simulink model "ManipulatorTrajectoryPlanning_Randomized"  (R2023b)
settings: Solver=VariableStepAuto  StartTime=0.0  StopTime=5  RelTol=1e-3
model workspace (MAT data in the model file):
  dq0 = [0; 0; 0; 0; 0; 0; 0; 0; 0]
  q0 = [0; 3.14159265359; 3.14159265359; 0; 0; 0; 0; 0; 0]
  robotToTest : robotics.RigidBodyTree (value not decoded)
symbols that are objects in the model workspace (value not decoded): robotToTest
undefined symbols (not defined in the file): X, Y, Z
libraries: sm_lib x140, nesl_utility x23, robotcorelib x1
(part 1 of 3)
settings Model: Creator=callie  LastModifiedBy=callie
settings OptimizationCC: ReuseModelBlockBuffer=off

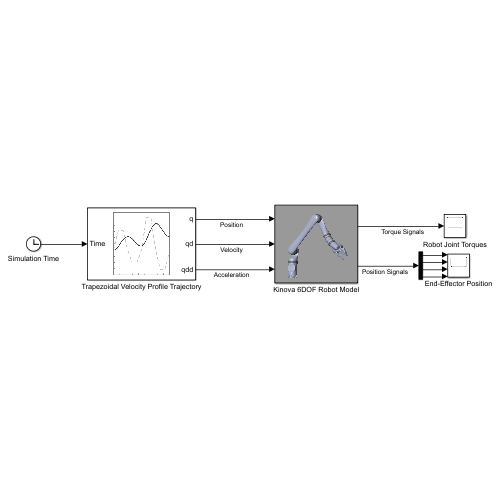
[thumbnail: Simulink's stored preview of the top-level diagram]
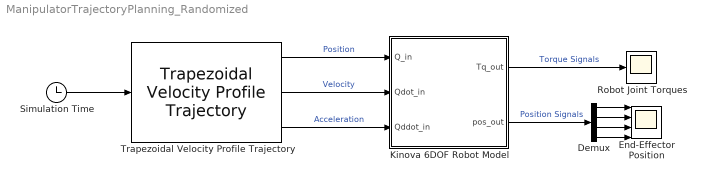
== system ManipulatorTrajectoryPlanning_Randomized ==
  Demux : Demux
  End-Effector Position : Scope  NumInputPorts=4
  Kinova 6DOF Robot Model : Subsystem
      mask Display: image('fullrobot.png'); % Use "Edit Image" on toolstrip to change.
  Robot Joint Torques : Scope
  Simulation Time : Clock
  Trapezoidal Velocity Profile Trajectory : robotcorelib/Trapezoidal Velocity Profile Trajectory  WaypointSource=Internal  Waypoints=[robotToTest.homeConfiguration robotToTest.randomConfiguration robotToTest.randomConfiguration]  NumParams=1  Parameter1=End Time  Parameter2=End Time  ParameterSource=Internal  PeakVelocity=[ 2; 2 ]  Acceleration=[ 1; 2 ]  EndTime=3  AccelTime=[ 1; 2 ]  SimulateUsing=Interpreted execution
  wires:
  Simulation Time/1 -> Trapezoidal Velocity Profile Trajectory/1
  Trapezoidal Velocity Profile Trajectory/1 -> Kinova 6DOF Robot Model/1(Q_in)  "Position"
  Trapezoidal Velocity Profile Trajectory/2 -> Kinova 6DOF Robot Model/2(Qdot_in)  "Velocity"
  Trapezoidal Velocity Profile Trajectory/3 -> Kinova 6DOF Robot Model/3(Qddot_in)  "Acceleration"
  Kinova 6DOF Robot Model/1(Tq_out) -> Robot Joint Torques/1  "Torque Signals"
  Kinova 6DOF Robot Model/2(pos_out) -> Demux/1  "Position Signals"
  Demux/1 -> End-Effector Position/1
  Demux/2 -> End-Effector Position/2
  Demux/3 -> End-Effector Position/3
  Demux/4 -> End-Effector Position/4

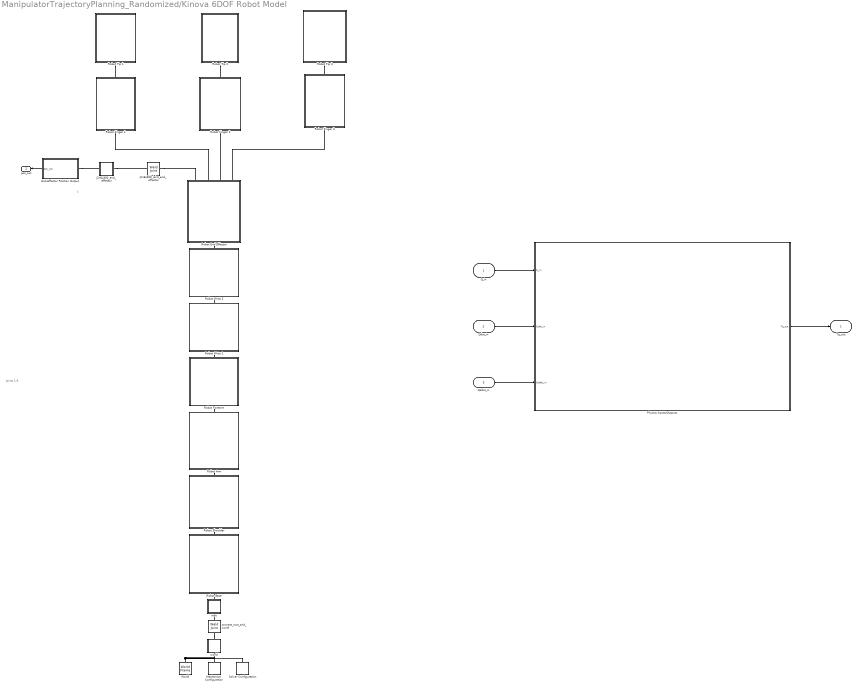
== system ManipulatorTrajectoryPlanning_Randomized/Kinova 6DOF Robot Model ==
  note: Joints 1-6
  note: {
  Q_in : Inport
  Qdot_in : Inport  Port=2
  Qddot_in : Inport  Port=3
  End-Effector Position Output : Subsystem
  Mechanism Configuration : sm_lib/Utilities/Mechanism Configuration  UniformGravity=Constant  GravityVector=[0, 0, 0]  GravityUnits=m/s^2  LinearizationDelta=0.001  JointModeTransitionNonlinearIterations=2
  Physics Inputs/Outputs : Subsystem
  Robot Tip 2 : Subsystem
      mask Display: image('fingerdistal2.png'); % Use "Edit Image" on toolstrip to change.
  Robot Finger 1 : Subsystem
      mask Display: image('fingerproximal1.png'); % Use "Edit Image" on toolstrip to change.
  Robot Finger 2 : Subsystem
      mask Display: image('fingerproximal2.png'); % Use "Edit Image" on toolstrip to change.
  Robot Finger 3 : Subsystem
      mask Display: image('fingerproximal3.png'); % Use "Edit Image" on toolstrip to change.
  Robot Tip 1 : Subsystem
      mask Display: image('fingerdistal1.png'); % Use "Edit Image" on toolstrip to change.
  Robot Tip 3 : Subsystem
      mask Display: image('fingerdistal3.png'); % Use "Edit Image" on toolstrip to change.
  Robot Arm : Subsystem
      mask Display: image('arm.png'); % Use "Edit Image" on toolstrip to change.
  Robot Base : Subsystem
      mask Display: image('Base.png'); % Use "Edit Image" on toolstrip to change.
  Robot End Effector : Subsystem
      mask Display: image('endeffector.png'); % Use "Edit Image" on toolstrip to change.
  Robot Forearm : Subsystem
      mask Display: image('forearm.png'); % Use "Edit Image" on toolstrip to change.
  Robot Shoulder : Subsystem
      mask Display: image('Shoulder.png'); % Use "Edit Image" on toolstrip to change.
  Robot Wrist 1 : Subsystem
      mask Display: image('wrist1.png'); % Use "Edit Image" on toolstrip to change.
  Robot Wrist 2 : Subsystem
      mask Display: image('wrist2.png'); % Use "Edit Image" on toolstrip to change.
  Solver Configuration : nesl_utility/Solver Configuration  PhysicalDomain=network_engine_domain  SubClassName=solver  LeftPortType=input  RightPortType=generic  Tones=[]  Harmonics=[]  SimulateNoise=off  Profile=off  UseLocalSampling=off  EnableSwitchedLinearOptims=on  FrequencyDomain=off  UseCCode=off  RelTol=0.001  AbsTol=0.001  MinStep=1e-09  ToWorkspace=off  RevertToSquareIcSolve=off  NumHomotopyIterations=100  PhasorMode=off  PhasorModeNumHarmonics=1  ConsistencySolver=NEWTON_XTOL_AFTER_FTOL  IndexReductionMethod=DerivativeReplacement  DoDC=off  ResidualTolerance=1e-09  ConsistencyTolSource=GLOBAL  ConsistencyAbsTol=0.001  ConsistencyRelTol=0.001  ConsistencyTolFactor=0.001  UseLocalSolver=off  LocalSolverChoice=NE_BACKWARD_EULER_ADVANCER  ResolveIndetEquations=on  FunctionEvalNumThread=1  LocalSolverSampleTime=0.001  DoFixedCost=off  MaxNonlinIter=3  MaxModeIter=2  ComputeImpulses=off  ImpulseIterations=2  LinearAlgebra=auto  LinearAlgebraNumThread=0  EquationFormulation=NE_TIME_EF  DelaysMemoryBudget=1024  AutomaticFiltering=on  FilteringTimeConstant=0.001  PartitionStorageMethod=AS_NEEDED  PartitionMemoryBudget=1024  PartitionMethod=ROBUST
  World : sm_lib/Frames and Transforms/World Frame
  connect_root_and_world : sm_lib/Joints/Weld Joint  JointMode=Normal  SenseConstraintForce=off  SenseConstraintForceX=off  SenseConstraintForceY=off  SenseConstraintForceZ=off  SenseConstraintTorque=off  SenseConstraintTorqueX=off  SenseConstraintTorqueY=off  SenseConstraintTorqueZ=off  SenseTotalForce=off  SenseTotalForceX=off  SenseTotalForceY=off  SenseTotalForceZ=off  SenseTotalTorque=off  SenseTotalTorqueX=off  SenseTotalTorqueY=off  SenseTotalTorqueZ=off  CompositeWrenchDir=FollowerOnBase  CompositeWrenchFrame=BaseFrame
  j2n6s300_end_effector : Subsystem
  j2n6s300_joint_end_effector : sm_lib/Joints/Weld Joint  JointMode=Normal  SenseConstraintForce=off  SenseConstraintForceX=off  SenseConstraintForceY=off  SenseConstraintForceZ=off  SenseConstraintTorque=off  SenseConstraintTorqueX=off  SenseConstraintTorqueY=off  SenseConstraintTorqueZ=off  SenseTotalForce=off  SenseTotalForceX=off  SenseTotalForceY=off  SenseTotalForceZ=off  SenseTotalTorque=off  SenseTotalTorqueX=off  SenseTotalTorqueY=off  SenseTotalTorqueZ=off  CompositeWrenchDir=FollowerOnBase  CompositeWrenchFrame=BaseFrame
  root : Subsystem
  world : Subsystem
  Tq_out : Outport
  pos_out : Outport  Port=2
  wires:
  Q_in/1 -> Physics Inputs/Outputs/1(Q_in)
  Physics Inputs/Outputs/1(Tq_out) -> Tq_out/1
  Qddot_in/1 -> Physics Inputs/Outputs/3(Qddot_in)
  Qdot_in/1 -> Physics Inputs/Outputs/2(Qdot_in)
  End-Effector Position Output/1(pos_out) -> pos_out/1
  connections:
  World/RConn1 -- Mechanism Configuration/RConn1 -- Solver Configuration/RConn1 -- world/LConn1
  connect_root_and_world/RConn1 -- root/LConn1
  j2n6s300_end_effector/LConn1 -- j2n6s300_joint_end_effector/RConn1
  connect_root_and_world/LConn1 -- world/RConn1
  Robot Base/LConn1 -- root/RConn1
  Robot Shoulder/LConn1 -- Robot Base/RConn1
  Robot Arm/LConn1 -- Robot Shoulder/RConn1
  Robot Forearm/LConn1 -- Robot Arm/RConn1
  Robot Wrist 1/LConn1 -- Robot Forearm/RConn1
  Robot Wrist 2/LConn1 -- Robot Wrist 1/RConn1
  Robot End Effector/LConn1 -- Robot Wrist 2/RConn1
  j2n6s300_joint_end_effector/LConn1 -- Robot End Effector/RConn1
  Robot Tip 1/LConn1 -- Robot Finger 1/RConn1
  Robot Finger 1/LConn1 -- Robot End Effector/RConn2
  Robot Tip 2/LConn1 -- Robot Finger 2/RConn1
  Robot Finger 2/LConn1 -- Robot End Effector/RConn3
  Robot Finger 3/LConn1 -- Robot End Effector/RConn4
  Robot Tip 3/LConn1 -- Robot Finger 3/RConn1
  End-Effector Position Output/LConn1 -- j2n6s300_end_effector/RConn1

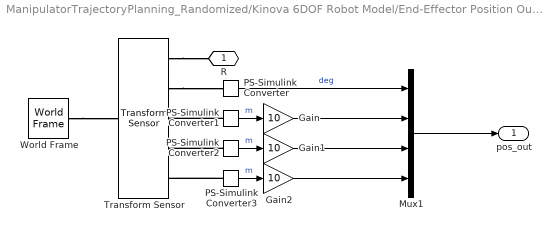
== system ManipulatorTrajectoryPlanning_Randomized/Kinova 6DOF Robot Model/End-Effector Position Output ==
  Gain : Gain  Gain=10
  Gain1 : Gain  Gain=10
  Gain2 : Gain  Gain=10
  Mux1 : Mux
  PS-Simulink Converter : nesl_utility/PS-Simulink Converter  PhysicalDomain=network_engine_domain  SubClassName=ps_output  LeftPortType=input  RightPortType=output  PseudoPeriodic=off  Frequencies=[]  VectorFormat=inherit  Unit=deg  AffineConversion=off
  PS-Simulink Converter1 : nesl_utility/PS-Simulink Converter  PhysicalDomain=network_engine_domain  SubClassName=ps_output  LeftPortType=input  RightPortType=output  PseudoPeriodic=off  Frequencies=[]  VectorFormat=inherit  Unit=m  AffineConversion=off
  PS-Simulink Converter2 : nesl_utility/PS-Simulink Converter  PhysicalDomain=network_engine_domain  SubClassName=ps_output  LeftPortType=input  RightPortType=output  PseudoPeriodic=off  Frequencies=[]  VectorFormat=inherit  Unit=m  AffineConversion=off
  PS-Simulink Converter3 : nesl_utility/PS-Simulink Converter  PhysicalDomain=network_engine_domain  SubClassName=ps_output  LeftPortType=input  RightPortType=output  PseudoPeriodic=off  Frequencies=[]  VectorFormat=inherit  Unit=m  AffineConversion=off
  Transform Sensor : sm_lib/Frames and Transforms/Transform Sensor  MeasurementFrame=World  SenseAngle=on  SenseAxis=off  SenseQ=off  SenseR=off  SenseRotationSequence=off  RotationSequence=XYX  SenseOmegaX=off  SenseOmegaY=off  SenseOmegaZ=off  SenseQDot=off  SenseRDot=off  SenseAlphaX=off  SenseAlphaY=off  SenseAlphaZ=off  SenseQDDot=off  SenseRDDot=off  SenseX=on  SenseY=on  SenseZ=on  SenseRad=off  SenseAzim=off  SenseDist=off  SenseInc=off  SenseXDot=off  SenseYDot=off  SenseZDot=off  SenseRadDot=off  SenseAzimDot=off  SenseDistDot=off  SenseIncDot=off  SenseXDDot=off  SenseYDDot=off  SenseZDDot=off  SenseRadDDot=off  SenseAzimDDot=off  SenseDistDDot=off  SenseIncDDot=off
  World Frame : sm_lib/Frames and Transforms/World Frame
  R : PMIOPort  Side=Left
  pos_out : Outport
  wires:
  PS-Simulink Converter/1 -> Mux1/1  "deg"
  PS-Simulink Converter3/1 -> Gain2/1  "m"
  PS-Simulink Converter2/1 -> Gain1/1  "m"
  PS-Simulink Converter1/1 -> Gain/1  "m"
  Mux1/1 -> pos_out/1
  Gain/1 -> Mux1/2
  Gain1/1 -> Mux1/3
  Gain2/1 -> Mux1/4
  connections:
  World Frame/RConn1 -- Transform Sensor/LConn1
  PS-Simulink Converter2/LConn1 -- Transform Sensor/RConn4
  Transform Sensor/RConn2 -- PS-Simulink Converter/LConn1
  PS-Simulink Converter3/LConn1 -- Transform Sensor/RConn5
  PS-Simulink Converter1/LConn1 -- Transform Sensor/RConn3
  Transform Sensor/RConn1 -- R/RConn1

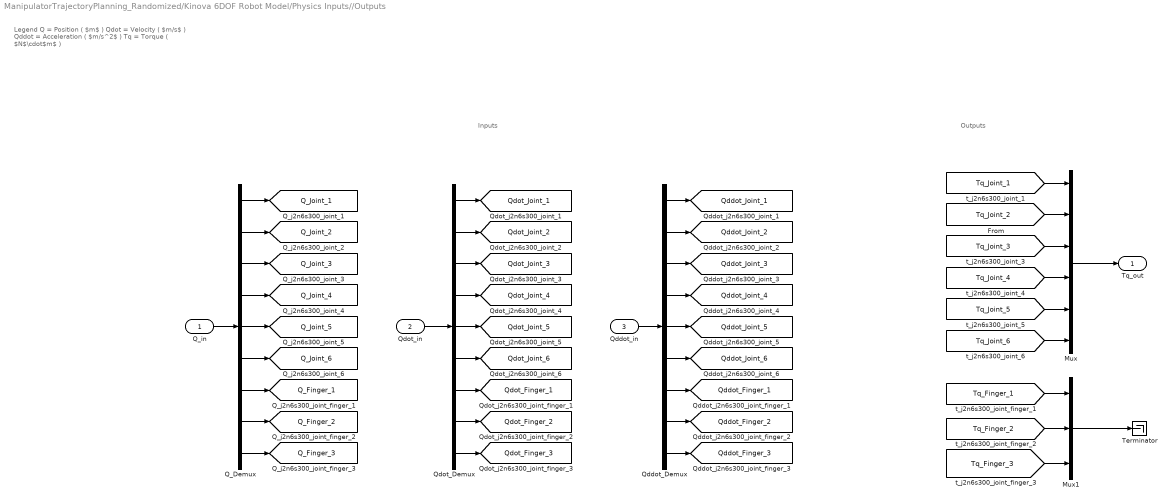
== system ManipulatorTrajectoryPlanning_Randomized/Kinova 6DOF Robot Model/Physics Inputs//Outputs ==
  note: Legend
      |
      | Q = Position ( $m$ )
      |
      | Qdot = Velocity ( $m/s$ )
      |
      | Qddot = Acceleration ( $m/s^2$ )
      |
      | Tq = Torque ( $N$\cdot$m$ )
  note: Inputs
  note: Outputs
  Q_in : Inport
  Qdot_in : Inport  Port=2
  Qddot_in : Inport  Port=3
  Mux : Mux  Inputs=6
  Mux1 : Mux  Inputs=3
  Q_Demux : Demux  Outputs=9
  Qddot_Demux : Demux  Outputs=9
  Qdot_Demux : Demux  Outputs=9
  Terminator : Terminator
  Tq_out : Outport
  tag scope: Q_Finger_1=global, Q_Finger_2=global, Q_Finger_3=global, Q_Joint_1=global, Q_Joint_2=global, Q_Joint_3=global, Q_Joint_4=global, Q_Joint_5=global, Q_Joint_6=global, Qddot_Finger_1=global, Qddot_Finger_2=global, Qddot_Finger_3=global, Qddot_Joint_1=global, Qddot_Joint_2=global, Qddot_Joint_3=global, Qddot_Joint_4=global, Qddot_Joint_5=global, Qddot_Joint_6=global, Qdot_Finger_1=global, Qdot_Finger_2=global, Qdot_Finger_3=global, Qdot_Joint_1=global, Qdot_Joint_2=global, Qdot_Joint_3=global, Qdot_Joint_4=global, Qdot_Joint_5=global, Qdot_Joint_6=global
  wires:
  Qdot_Demux/2 -> [Qdot_Joint_2]
  Qddot_Demux/2 -> [Qddot_Joint_2]
  Qdot_Demux/4 -> [Qdot_Joint_4]
  Qdot_Demux/6 -> [Qdot_Joint_6]
  Q_in/1 -> Q_Demux/1
  Q_Demux/4 -> [Q_Joint_4]
  Qdot_in/1 -> Qdot_Demux/1
  Qdot_Demux/8 -> [Qdot_Finger_2]
  Q_Demux/8 -> [Q_Finger_2]
  Q_Demux/5 -> [Q_Joint_5]
  Q_Demux/6 -> [Q_Joint_6]
  Qdot_Demux/7 -> [Qdot_Finger_1]
  Qddot_Demux/6 -> [Qddot_Joint_6]
  Q_Demux/9 -> [Q_Finger_3]
  Qddot_Demux/5 -> [Qddot_Joint_5]
  Qdot_Demux/1 -> [Qdot_Joint_1]
  Qdot_Demux/9 -> [Qdot_Finger_3]
  Qdot_Demux/5 -> [Qdot_Joint_5]
  Qddot_Demux/3 -> [Qddot_Joint_3]
  Qddot_Demux/7 -> [Qddot_Finger_1]
  Q_Demux/1 -> [Q_Joint_1]
  Qdot_Demux/3 -> [Qdot_Joint_3]
  Q_Demux/3 -> [Q_Joint_3]
  Qddot_Demux/1 -> [Qddot_Joint_1]
  Q_Demux/2 -> [Q_Joint_2]
  Qddot_Demux/4 -> [Qddot_Joint_4]
  Qddot_in/1 -> Qddot_Demux/1
  Q_Demux/7 -> [Q_Finger_1]
  Qddot_Demux/9 -> [Qddot_Finger_3]
  Qddot_Demux/8 -> [Qddot_Finger_2]
  [Tq_Joint_6] -> Mux/6
  [Tq_Finger_3] -> Mux1/3
  [Tq_Joint_3] -> Mux/3
  [Tq_Joint_2] -> Mux/2
  [Tq_Finger_2] -> Mux1/2
  [Tq_Finger_1] -> Mux1/1
  [Tq_Joint_1] -> Mux/1
  Mux/1 -> Tq_out/1
  [Tq_Joint_5] -> Mux/5
  Mux1/1 -> Terminator/1
  [Tq_Joint_4] -> Mux/4

== system ManipulatorTrajectoryPlanning_Randomized/Kinova 6DOF Robot Model/Robot Tip 2 ==
  j2n6s300_joint_finger_tip_2 : sm_lib/Joints/Weld Joint  JointMode=Normal  SenseConstraintForce=off  SenseConstraintForceX=off  SenseConstraintForceY=off  SenseConstraintForceZ=off  SenseConstraintTorque=off  SenseConstraintTorqueX=off  SenseConstraintTorqueY=off  SenseConstraintTorqueZ=off  SenseTotalForce=off  SenseTotalForceX=off  SenseTotalForceY=off  SenseTotalForceZ=off  SenseTotalTorque=off  SenseTotalTorqueX=off  SenseTotalTorqueY=off  SenseTotalTorqueZ=off  CompositeWrenchDir=FollowerOnBase  CompositeWrenchFrame=BaseFrame
  j2n6s300_link_finger_tip_2 : Subsystem
  Conn1 : PMIOPort  Side=Left
  connections:
  j2n6s300_joint_finger_tip_2/RConn1 -- j2n6s300_link_finger_tip_2/LConn1
  j2n6s300_joint_finger_tip_2/LConn1 -- Conn1/RConn1

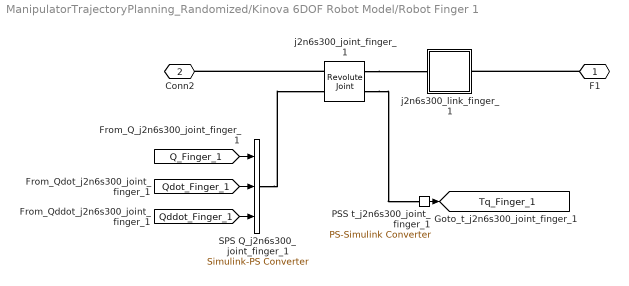
== system ManipulatorTrajectoryPlanning_Randomized/Kinova 6DOF Robot Model/Robot Finger 1 ==
  PSS t_j2n6s300_joint_finger_1 : nesl_utility/PS-Simulink Converter  PhysicalDomain=network_engine_domain  SubClassName=ps_output  LeftPortType=input  RightPortType=output  PseudoPeriodic=off  Frequencies=[]  VectorFormat=inherit  Unit=inherit  AffineConversion=off
  SPS Q_j2n6s300_joint_finger_1 : nesl_utility/Simulink-PS Converter  PhysicalDomain=network_engine_domain  SubClassName=ps_input  LeftPortType=input  RightPortType=output  PseudoPeriodic=off  Frequencies=[]  NoiseDistribution=none  NoiseParameters=[]  Unit=1  AffineConversion=off  FilteringAndDerivatives=provide  SimscapeFilterOrder=1  InputFilterTimeConstant=0.001  UdotUserProvided=2
  j2n6s300_joint_finger_1 : sm_lib/Joints/Revolute Joint  JointMode=Normal  SenseConstraintForce=off  SenseConstraintForceX=off  SenseConstraintForceY=off  SenseConstraintForceZ=off  SenseConstraintTorque=off  SenseConstraintTorqueX=off  SenseConstraintTorqueY=off  SenseConstraintTorqueZ=off  SenseTotalForce=off  SenseTotalForceX=off  SenseTotalForceY=off  SenseTotalForceZ=off  SenseTotalTorque=off  SenseTotalTorqueX=off  SenseTotalTorqueY=off  SenseTotalTorqueZ=off  CompositeWrenchDir=FollowerOnBase  CompositeWrenchFrame=BaseFrame  EquilibriumPosition=0  EquilibriumPositionUnits=deg  SpringStiffness=0  SpringStiffnessUnits=N*m/deg  DampingCoefficient=0  DampingCoefficientUnits=kg*m^2/(rad*s)  TorqueActuationMode=ComputedTorque  MotionActuationMode=InputMotion  SensePosition=off  SenseVelocity=off  SenseAcceleration=off  SenseTorqueForce=on  SenseLowerLimitTorqueForce=off  SenseUpperLimitTorqueForce=off  LowerLimitSpecify=on  LowerLimitBound=0  LowerLimitBoundUnits=rad  LowerLimitStiffness=1e4  LowerLimitStiffnessUnits=N*m/deg  LowerLimitDamping=10  LowerLimitDampingUnits=N*m/(deg/s)  LowerLimitTransitionRegionWidth=0.1  LowerLimitTransitionRegionWidthUnits=deg  UpperLimitSpecify=on  UpperLimitBound=2  UpperLimitBoundUnits=rad  UpperLimitStiffness=1e4  UpperLimitStiffnessUnits=N*m/deg  UpperLimitDamping=10  UpperLimitDampingUnits=N*m/(deg/s)  UpperLimitTransitionRegionWidth=0.1  UpperLimitTransitionRegionWidthUnits=deg  PositionTargetSpecify=on  PositionTargetPriority=High  PositionTargetValue=q0(7)  PositionTargetValueUnits=rad  VelocityTargetSpecify=on  VelocityTargetPriority=High  VelocityTargetValue=dq0(7)  VelocityTargetValueUnits=rad/s
  j2n6s300_link_finger_1 : Subsystem
  F1 : PMIOPort  Side=Right
  Conn2 : PMIOPort  Port=2  Side=Left
  tag scope: Tq_Finger_1=global
  wires:
  [Qddot_Finger_1] -> SPS Q_j2n6s300_joint_finger_1/3
  [Qdot_Finger_1] -> SPS Q_j2n6s300_joint_finger_1/2
  PSS t_j2n6s300_joint_finger_1/1 -> [Tq_Finger_1]
  [Q_Finger_1] -> SPS Q_j2n6s300_joint_finger_1/1
  connections:
  j2n6s300_joint_finger_1/LConn1 -- Conn2/RConn1
  j2n6s300_joint_finger_1/RConn1 -- j2n6s300_link_finger_1/LConn1
  j2n6s300_joint_finger_1/RConn2 -- PSS t_j2n6s300_joint_finger_1/LConn1
  SPS Q_j2n6s300_joint_finger_1/RConn1 -- j2n6s300_joint_finger_1/LConn2
  F1/RConn1 -- j2n6s300_link_finger_1/RConn1

== system ManipulatorTrajectoryPlanning_Randomized/Kinova 6DOF Robot Model/Robot Finger 2 ==
  PSS t_j2n6s300_joint_finger_2 : nesl_utility/PS-Simulink Converter  PhysicalDomain=network_engine_domain  SubClassName=ps_output  LeftPortType=input  RightPortType=output  PseudoPeriodic=off  Frequencies=[]  VectorFormat=inherit  Unit=inherit  AffineConversion=off
  SPS Q_j2n6s300_joint_finger_2 : nesl_utility/Simulink-PS Converter  PhysicalDomain=network_engine_domain  SubClassName=ps_input  LeftPortType=input  RightPortType=output  PseudoPeriodic=off  Frequencies=[]  NoiseDistribution=none  NoiseParameters=[]  Unit=1  AffineConversion=off  FilteringAndDerivatives=provide  SimscapeFilterOrder=1  InputFilterTimeConstant=0.001  UdotUserProvided=2
  j2n6s300_joint_finger_2 : sm_lib/Joints/Revolute Joint  JointMode=Normal  SenseConstraintForce=off  SenseConstraintForceX=off  SenseConstraintForceY=off  SenseConstraintForceZ=off  SenseConstraintTorque=off  SenseConstraintTorqueX=off  SenseConstraintTorqueY=off  SenseConstraintTorqueZ=off  SenseTotalForce=off  SenseTotalForceX=off  SenseTotalForceY=off  SenseTotalForceZ=off  SenseTotalTorque=off  SenseTotalTorqueX=off  SenseTotalTorqueY=off  SenseTotalTorqueZ=off  CompositeWrenchDir=FollowerOnBase  CompositeWrenchFrame=BaseFrame  EquilibriumPosition=0  EquilibriumPositionUnits=deg  SpringStiffness=0  SpringStiffnessUnits=N*m/deg  DampingCoefficient=0  DampingCoefficientUnits=kg*m^2/(rad*s)  TorqueActuationMode=ComputedTorque  MotionActuationMode=InputMotion  SensePosition=off  SenseVelocity=off  SenseAcceleration=off  SenseTorqueForce=on  SenseLowerLimitTorqueForce=off  SenseUpperLimitTorqueForce=off  LowerLimitSpecify=on  LowerLimitBound=0  LowerLimitBoundUnits=rad  LowerLimitStiffness=1e4  LowerLimitStiffnessUnits=N*m/deg  LowerLimitDamping=10  LowerLimitDampingUnits=N*m/(deg/s)  LowerLimitTransitionRegionWidth=0.1  LowerLimitTransitionRegionWidthUnits=deg  UpperLimitSpecify=on  UpperLimitBound=2  UpperLimitBoundUnits=rad  UpperLimitStiffness=1e4  UpperLimitStiffnessUnits=N*m/deg  UpperLimitDamping=10  UpperLimitDampingUnits=N*m/(deg/s)  UpperLimitTransitionRegionWidth=0.1  UpperLimitTransitionRegionWidthUnits=deg  PositionTargetSpecify=on  PositionTargetPriority=High  PositionTargetValue=q0(8)  PositionTargetValueUnits=rad  VelocityTargetSpecify=on  VelocityTargetPriority=High  VelocityTargetValue=dq0(8)  VelocityTargetValueUnits=rad/s
  j2n6s300_link_finger_2 : Subsystem
  F1 : PMIOPort  Side=Right
  Conn2 : PMIOPort  Port=2  Side=Left
  tag scope: Tq_Finger_2=global
  wires:
  [Qddot_Finger_2] -> SPS Q_j2n6s300_joint_finger_2/3
  PSS t_j2n6s300_joint_finger_2/1 -> [Tq_Finger_2]
  [Qdot_Finger_2] -> SPS Q_j2n6s300_joint_finger_2/2
  [Q_Finger_2] -> SPS Q_j2n6s300_joint_finger_2/1
  connections:
  F1/RConn1 -- j2n6s300_link_finger_2/RConn1
  j2n6s300_joint_finger_2/RConn2 -- PSS t_j2n6s300_joint_finger_2/LConn1
  j2n6s300_joint_finger_2/RConn1 -- j2n6s300_link_finger_2/LConn1
  SPS Q_j2n6s300_joint_finger_2/RConn1 -- j2n6s300_joint_finger_2/LConn2
  j2n6s300_joint_finger_2/LConn1 -- Conn2/RConn1

== system ManipulatorTrajectoryPlanning_Randomized/Kinova 6DOF Robot Model/Robot Finger 3 ==
  PSS t_j2n6s300_joint_finger_3 : nesl_utility/PS-Simulink Converter  PhysicalDomain=network_engine_domain  SubClassName=ps_output  LeftPortType=input  RightPortType=output  PseudoPeriodic=off  Frequencies=[]  VectorFormat=inherit  Unit=inherit  AffineConversion=off
  SPS Q_j2n6s300_joint_finger_3 : nesl_utility/Simulink-PS Converter  PhysicalDomain=network_engine_domain  SubClassName=ps_input  LeftPortType=input  RightPortType=output  PseudoPeriodic=off  Frequencies=[]  NoiseDistribution=none  NoiseParameters=[]  Unit=1  AffineConversion=off  FilteringAndDerivatives=provide  SimscapeFilterOrder=1  InputFilterTimeConstant=0.001  UdotUserProvided=2
  j2n6s300_joint_finger_3 : sm_lib/Joints/Revolute Joint  JointMode=Normal  SenseConstraintForce=off  SenseConstraintForceX=off  SenseConstraintForceY=off  SenseConstraintForceZ=off  SenseConstraintTorque=off  SenseConstraintTorqueX=off  SenseConstraintTorqueY=off  SenseConstraintTorqueZ=off  SenseTotalForce=off  SenseTotalForceX=off  SenseTotalForceY=off  SenseTotalForceZ=off  SenseTotalTorque=off  SenseTotalTorqueX=off  SenseTotalTorqueY=off  SenseTotalTorqueZ=off  CompositeWrenchDir=FollowerOnBase  CompositeWrenchFrame=BaseFrame  EquilibriumPosition=0  EquilibriumPositionUnits=deg  SpringStiffness=0  SpringStiffnessUnits=N*m/deg  DampingCoefficient=0  DampingCoefficientUnits=kg*m^2/(rad*s)  TorqueActuationMode=ComputedTorque  MotionActuationMode=InputMotion  SensePosition=off  SenseVelocity=off  SenseAcceleration=off  SenseTorqueForce=on  SenseLowerLimitTorqueForce=off  SenseUpperLimitTorqueForce=off  LowerLimitSpecify=on  LowerLimitBound=0  LowerLimitBoundUnits=rad  LowerLimitStiffness=1e4  LowerLimitStiffnessUnits=N*m/deg  LowerLimitDamping=10  LowerLimitDampingUnits=N*m/(deg/s)  LowerLimitTransitionRegionWidth=0.1  LowerLimitTransitionRegionWidthUnits=deg  UpperLimitSpecify=on  UpperLimitBound=2  UpperLimitBoundUnits=rad  UpperLimitStiffness=1e4  UpperLimitStiffnessUnits=N*m/deg  UpperLimitDamping=10  UpperLimitDampingUnits=N*m/(deg/s)  UpperLimitTransitionRegionWidth=0.1  UpperLimitTransitionRegionWidthUnits=deg  PositionTargetSpecify=on  PositionTargetPriority=High  PositionTargetValue=q0(9)  PositionTargetValueUnits=rad  VelocityTargetSpecify=on  VelocityTargetPriority=High  VelocityTargetValue=dq0(9)  VelocityTargetValueUnits=rad/s
  j2n6s300_link_finger_3 : Subsystem
  F1 : PMIOPort  Side=Right
  Conn1 : PMIOPort  Port=2  Side=Left
  tag scope: Tq_Finger_3=global
  wires:
  PSS t_j2n6s300_joint_finger_3/1 -> [Tq_Finger_3]
  [Qddot_Finger_3] -> SPS Q_j2n6s300_joint_finger_3/3
  [Q_Finger_3] -> SPS Q_j2n6s300_joint_finger_3/1
  [Qdot_Finger_3] -> SPS Q_j2n6s300_joint_finger_3/2
  connections:
  F1/RConn1 -- j2n6s300_link_finger_3/RConn1
  j2n6s300_joint_finger_3/RConn2 -- PSS t_j2n6s300_joint_finger_3/LConn1
  SPS Q_j2n6s300_joint_finger_3/RConn1 -- j2n6s300_joint_finger_3/LConn2
  j2n6s300_joint_finger_3/RConn1 -- j2n6s300_link_finger_3/LConn1
  j2n6s300_joint_finger_3/LConn1 -- Conn1/RConn1

== system ManipulatorTrajectoryPlanning_Randomized/Kinova 6DOF Robot Model/Robot Tip 1 ==
  j2n6s300_joint_finger_tip_1 : sm_lib/Joints/Weld Joint  JointMode=Normal  SenseConstraintForce=off  SenseConstraintForceX=off  SenseConstraintForceY=off  SenseConstraintForceZ=off  SenseConstraintTorque=off  SenseConstraintTorqueX=off  SenseConstraintTorqueY=off  SenseConstraintTorqueZ=off  SenseTotalForce=off  SenseTotalForceX=off  SenseTotalForceY=off  SenseTotalForceZ=off  SenseTotalTorque=off  SenseTotalTorqueX=off  SenseTotalTorqueY=off  SenseTotalTorqueZ=off  CompositeWrenchDir=FollowerOnBase  CompositeWrenchFrame=BaseFrame
  j2n6s300_link_finger_tip_1 : Subsystem
  Conn1 : PMIOPort  Side=Left
  connections:
  j2n6s300_joint_finger_tip_1/RConn1 -- j2n6s300_link_finger_tip_1/LConn1
  j2n6s300_joint_finger_tip_1/LConn1 -- Conn1/RConn1

== system ManipulatorTrajectoryPlanning_Randomized/Kinova 6DOF Robot Model/Robot Tip 3 ==
  j2n6s300_joint_finger_tip_3 : sm_lib/Joints/Weld Joint  JointMode=Normal  SenseConstraintForce=off  SenseConstraintForceX=off  SenseConstraintForceY=off  SenseConstraintForceZ=off  SenseConstraintTorque=off  SenseConstraintTorqueX=off  SenseConstraintTorqueY=off  SenseConstraintTorqueZ=off  SenseTotalForce=off  SenseTotalForceX=off  SenseTotalForceY=off  SenseTotalForceZ=off  SenseTotalTorque=off  SenseTotalTorqueX=off  SenseTotalTorqueY=off  SenseTotalTorqueZ=off  CompositeWrenchDir=FollowerOnBase  CompositeWrenchFrame=BaseFrame
  j2n6s300_link_finger_tip_3 : Subsystem
  Conn1 : PMIOPort  Side=Left
  connections:
  j2n6s300_joint_finger_tip_3/LConn1 -- Conn1/RConn1
  j2n6s300_joint_finger_tip_3/RConn1 -- j2n6s300_link_finger_tip_3/LConn1

== system ManipulatorTrajectoryPlanning_Randomized/Kinova 6DOF Robot Model/Robot Arm ==
  PSS t_j2n6s300_joint_2 : nesl_utility/PS-Simulink Converter  PhysicalDomain=network_engine_domain  SubClassName=ps_output  LeftPortType=input  RightPortType=output  PseudoPeriodic=off  Frequencies=[]  VectorFormat=inherit  Unit=inherit  AffineConversion=off
  SPS Q_j2n6s300_joint_2 : nesl_utility/Simulink-PS Converter  PhysicalDomain=network_engine_domain  SubClassName=ps_input  LeftPortType=input  RightPortType=output  PseudoPeriodic=off  Frequencies=[]  NoiseDistribution=none  NoiseParameters=[]  Unit=1  AffineConversion=off  FilteringAndDerivatives=provide  SimscapeFilterOrder=1  InputFilterTimeConstant=0.001  UdotUserProvided=2
  j2n6s300_joint_2 : sm_lib/Joints/Revolute Joint  JointMode=Normal  SenseConstraintForce=off  SenseConstraintForceX=off  SenseConstraintForceY=off  SenseConstraintForceZ=off  SenseConstraintTorque=off  SenseConstraintTorqueX=off  SenseConstraintTorqueY=off  SenseConstraintTorqueZ=off  SenseTotalForce=off  SenseTotalForceX=off  SenseTotalForceY=off  SenseTotalForceZ=off  SenseTotalTorque=off  SenseTotalTorqueX=off  SenseTotalTorqueY=off  SenseTotalTorqueZ=off  CompositeWrenchDir=FollowerOnBase  CompositeWrenchFrame=BaseFrame  EquilibriumPosition=0  EquilibriumPositionUnits=deg  SpringStiffness=0  SpringStiffnessUnits=N*m/deg  DampingCoefficient=0  DampingCoefficientUnits=kg*m^2/(rad*s)  TorqueActuationMode=ComputedTorque  MotionActuationMode=InputMotion  SensePosition=off  SenseVelocity=off  SenseAcceleration=off  SenseTorqueForce=on  SenseLowerLimitTorqueForce=off  SenseUpperLimitTorqueForce=off  LowerLimitSpecify=on  LowerLimitBound=0.820304748437  LowerLimitBoundUnits=rad  LowerLimitStiffness=1e4  LowerLimitStiffnessUnits=N*m/deg  LowerLimitDamping=10  LowerLimitDampingUnits=N*m/(deg/s)  LowerLimitTransitionRegionWidth=0.1  LowerLimitTransitionRegionWidthUnits=deg  UpperLimitSpecify=on  UpperLimitBound=5.46288055874  UpperLimitBoundUnits=rad  UpperLimitStiffness=1e4  UpperLimitStiffnessUnits=N*m/deg  UpperLimitDamping=10  UpperLimitDampingUnits=N*m/(deg/s)  UpperLimitTransitionRegionWidth=0.1  UpperLimitTransitionRegionWidthUnits=deg  PositionTargetSpecify=on  PositionTargetPriority=High  PositionTargetValue=q0(2)  PositionTargetValueUnits=rad  VelocityTargetSpecify=on  VelocityTargetPriority=High  VelocityTargetValue=dq0(2)  VelocityTargetValueUnits=rad/s
  j2n6s300_link_2 : Subsystem
  Robot Forearm : PMIOPort  Side=Right
  Robot Shoulder : PMIOPort  Port=2  Side=Left
  tag scope: Tq_Joint_2=global
  wires:
  PSS t_j2n6s300_joint_2/1 -> [Tq_Joint_2]
  [Q_Joint_2] -> SPS Q_j2n6s300_joint_2/1
  [Qdot_Joint_2] -> SPS Q_j2n6s300_joint_2/2
  [Qddot_Joint_2] -> SPS Q_j2n6s300_joint_2/3
  connections:
  j2n6s300_joint_2/RConn2 -- PSS t_j2n6s300_joint_2/LConn1
  j2n6s300_joint_2/RConn1 -- j2n6s300_link_2/LConn1
  SPS Q_j2n6s300_joint_2/RConn1 -- j2n6s300_joint_2/LConn2
  j2n6s300_joint_2/LConn1 -- Robot Shoulder/RConn1
  Robot Forearm/RConn1 -- j2n6s300_link_2/RConn1

== system ManipulatorTrajectoryPlanning_Randomized/Kinova 6DOF Robot Model/Robot Base ==
  j2n6s300_joint_base : sm_lib/Joints/Weld Joint  JointMode=Normal  SenseConstraintForce=off  SenseConstraintForceX=off  SenseConstraintForceY=off  SenseConstraintForceZ=off  SenseConstraintTorque=off  SenseConstraintTorqueX=off  SenseConstraintTorqueY=off  SenseConstraintTorqueZ=off  SenseTotalForce=off  SenseTotalForceX=off  SenseTotalForceY=off  SenseTotalForceZ=off  SenseTotalTorque=off  SenseTotalTorqueX=off  SenseTotalTorqueY=off  SenseTotalTorqueZ=off  CompositeWrenchDir=FollowerOnBase  CompositeWrenchFrame=BaseFrame
  j2n6s300_link_base : Subsystem
  Robot Shoulder : PMIOPort  Side=Right
  Root : PMIOPort  Port=2  Side=Left
  connections:
  j2n6s300_joint_base/RConn1 -- j2n6s300_link_base/LConn1
  Root/RConn1 -- j2n6s300_joint_base/LConn1
  j2n6s300_link_base/RConn1 -- Robot Shoulder/RConn1

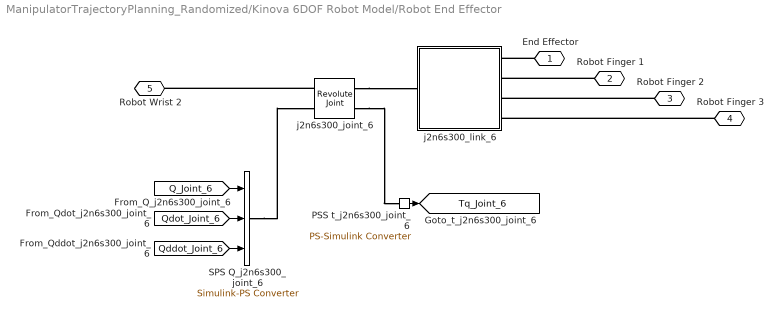
== system ManipulatorTrajectoryPlanning_Randomized/Kinova 6DOF Robot Model/Robot End Effector ==
  PSS t_j2n6s300_joint_6 : nesl_utility/PS-Simulink Converter  PhysicalDomain=network_engine_domain  SubClassName=ps_output  LeftPortType=input  RightPortType=output  PseudoPeriodic=off  Frequencies=[]  VectorFormat=inherit  Unit=inherit  AffineConversion=off
  SPS Q_j2n6s300_joint_6 : nesl_utility/Simulink-PS Converter  PhysicalDomain=network_engine_domain  SubClassName=ps_input  LeftPortType=input  RightPortType=output  PseudoPeriodic=off  Frequencies=[]  NoiseDistribution=none  NoiseParameters=[]  Unit=1  AffineConversion=off  FilteringAndDerivatives=provide  SimscapeFilterOrder=1  InputFilterTimeConstant=0.001  UdotUserProvided=2
  j2n6s300_joint_6 : sm_lib/Joints/Revolute Joint  JointMode=Normal  SenseConstraintForce=off  SenseConstraintForceX=off  SenseConstraintForceY=off  SenseConstraintForceZ=off  SenseConstraintTorque=off  SenseConstraintTorqueX=off  SenseConstraintTorqueY=off  SenseConstraintTorqueZ=off  SenseTotalForce=off  SenseTotalForceX=off  SenseTotalForceY=off  SenseTotalForceZ=off  SenseTotalTorque=off  SenseTotalTorqueX=off  SenseTotalTorqueY=off  SenseTotalTorqueZ=off  CompositeWrenchDir=FollowerOnBase  CompositeWrenchFrame=BaseFrame  EquilibriumPosition=0  EquilibriumPositionUnits=deg  SpringStiffness=0  SpringStiffnessUnits=N*m/deg  DampingCoefficient=0  DampingCoefficientUnits=kg*m^2/(rad*s)  TorqueActuationMode=ComputedTorque  MotionActuationMode=InputMotion  SensePosition=off  SenseVelocity=off  SenseAcceleration=off  SenseTorqueForce=on  SenseLowerLimitTorqueForce=off  SenseUpperLimitTorqueForce=off  LowerLimitSpecify=off  LowerLimitBound=-90  LowerLimitBoundUnits=deg  LowerLimitStiffness=1e4  LowerLimitStiffnessUnits=N*m/deg  LowerLimitDamping=10  LowerLimitDampingUnits=N*m/(deg/s)  LowerLimitTransitionRegionWidth=0.1  LowerLimitTransitionRegionWidthUnits=deg  UpperLimitSpecify=off  UpperLimitBound=90  UpperLimitBoundUnits=deg  UpperLimitStiffness=1e4  UpperLimitStiffnessUnits=N*m/deg  UpperLimitDamping=10  UpperLimitDampingUnits=N*m/(deg/s)  UpperLimitTransitionRegionWidth=0.1  UpperLimitTransitionRegionWidthUnits=deg  PositionTargetSpecify=on  PositionTargetPriority=High  PositionTargetValue=q0(6)  PositionTargetValueUnits=rad  VelocityTargetSpecify=on  VelocityTargetPriority=High  VelocityTargetValue=dq0(6)  VelocityTargetValueUnits=rad/s
  j2n6s300_link_6 : Subsystem
  End Effector : PMIOPort  Side=Right
  Robot Finger 1 : PMIOPort  Port=2  Side=Right
  Robot Finger 2 : PMIOPort  Port=3  Side=Right
  Robot Finger 3 : PMIOPort  Port=4  Side=Right
  Robot Wrist 2 : PMIOPort  Port=5  Side=Left
  tag scope: Tq_Joint_6=global
  wires:
  [Qdot_Joint_6] -> SPS Q_j2n6s300_joint_6/2
  [Qddot_Joint_6] -> SPS Q_j2n6s300_joint_6/3
  PSS t_j2n6s300_joint_6/1 -> [Tq_Joint_6]
  [Q_Joint_6] -> SPS Q_j2n6s300_joint_6/1
  connections:
  Robot Finger 2/RConn1 -- j2n6s300_link_6/RConn3
  Robot Finger 1/RConn1 -- j2n6s300_link_6/RConn2
  j2n6s300_joint_6/RConn2 -- PSS t_j2n6s300_joint_6/LConn1
  SPS Q_j2n6s300_joint_6/RConn1 -- j2n6s300_joint_6/LConn2
  j2n6s300_joint_6/RConn1 -- j2n6s300_link_6/LConn1
  Robot Finger 3/RConn1 -- j2n6s300_link_6/RConn4
  End Effector/RConn1 -- j2n6s300_link_6/RConn1
  j2n6s300_joint_6/LConn1 -- Robot Wrist 2/RConn1

== system ManipulatorTrajectoryPlanning_Randomized/Kinova 6DOF Robot Model/Robot Forearm ==
  PSS t_j2n6s300_joint_3 : nesl_utility/PS-Simulink Converter  PhysicalDomain=network_engine_domain  SubClassName=ps_output  LeftPortType=input  RightPortType=output  PseudoPeriodic=off  Frequencies=[]  VectorFormat=inherit  Unit=inherit  AffineConversion=off
  SPS Q_j2n6s300_joint_3 : nesl_utility/Simulink-PS Converter  PhysicalDomain=network_engine_domain  SubClassName=ps_input  LeftPortType=input  RightPortType=output  PseudoPeriodic=off  Frequencies=[]  NoiseDistribution=none  NoiseParameters=[]  Unit=1  AffineConversion=off  FilteringAndDerivatives=provide  SimscapeFilterOrder=1  InputFilterTimeConstant=0.001  UdotUserProvided=2
  j2n6s300_joint_3 : sm_lib/Joints/Revolute Joint  JointMode=Normal  SenseConstraintForce=off  SenseConstraintForceX=off  SenseConstraintForceY=off  SenseConstraintForceZ=off  SenseConstraintTorque=off  SenseConstraintTorqueX=off  SenseConstraintTorqueY=off  SenseConstraintTorqueZ=off  SenseTotalForce=off  SenseTotalForceX=off  SenseTotalForceY=off  SenseTotalForceZ=off  SenseTotalTorque=off  SenseTotalTorqueX=off  SenseTotalTorqueY=off  SenseTotalTorqueZ=off  CompositeWrenchDir=FollowerOnBase  CompositeWrenchFrame=BaseFrame  EquilibriumPosition=0  EquilibriumPositionUnits=deg  SpringStiffness=0  SpringStiffnessUnits=N*m/deg  DampingCoefficient=0  DampingCoefficientUnits=kg*m^2/(rad*s)  TorqueActuationMode=ComputedTorque  MotionActuationMode=InputMotion  SensePosition=off  SenseVelocity=off  SenseAcceleration=off  SenseTorqueForce=on  SenseLowerLimitTorqueForce=off  SenseUpperLimitTorqueForce=off  LowerLimitSpecify=on  LowerLimitBound=0.331612557879  LowerLimitBoundUnits=rad  LowerLimitStiffness=1e4  LowerLimitStiffnessUnits=N*m/deg  LowerLimitDamping=10  LowerLimitDampingUnits=N*m/(deg/s)  LowerLimitTransitionRegionWidth=0.1  LowerLimitTransitionRegionWidthUnits=deg  UpperLimitSpecify=on  UpperLimitBound=5.9515727493  UpperLimitBoundUnits=rad  UpperLimitStiffness=1e4  UpperLimitStiffnessUnits=N*m/deg  UpperLimitDamping=10  UpperLimitDampingUnits=N*m/(deg/s)  UpperLimitTransitionRegionWidth=0.1  UpperLimitTransitionRegionWidthUnits=deg  PositionTargetSpecify=on  PositionTargetPriority=High  PositionTargetValue=q0(3)  PositionTargetValueUnits=rad  VelocityTargetSpecify=on  VelocityTargetPriority=High  VelocityTargetValue=dq0(3)  VelocityTargetValueUnits=rad/s
  j2n6s300_link_3 : Subsystem
  Robot Wrist 1 : PMIOPort  Side=Right
  Robot Arm : PMIOPort  Port=2  Side=Left
  tag scope: Tq_Joint_3=global
  wires:
  [Q_Joint_3] -> SPS Q_j2n6s300_joint_3/1
  [Qddot_Joint_3] -> SPS Q_j2n6s300_joint_3/3
  [Qdot_Joint_3] -> SPS Q_j2n6s300_joint_3/2
  PSS t_j2n6s300_joint_3/1 -> [Tq_Joint_3]
  connections:
  j2n6s300_joint_3/RConn2 -- PSS t_j2n6s300_joint_3/LConn1
  j2n6s300_joint_3/RConn1 -- j2n6s300_link_3/LConn1
  SPS Q_j2n6s300_joint_3/RConn1 -- j2n6s300_joint_3/LConn2
  j2n6s300_joint_3/LConn1 -- Robot Arm/RConn1
  Robot Wrist 1/RConn1 -- j2n6s300_link_3/RConn1

== system ManipulatorTrajectoryPlanning_Randomized/Kinova 6DOF Robot Model/Robot Shoulder ==
  PSS t_j2n6s300_joint_1 : nesl_utility/PS-Simulink Converter  PhysicalDomain=network_engine_domain  SubClassName=ps_output  LeftPortType=input  RightPortType=output  PseudoPeriodic=off  Frequencies=[]  VectorFormat=inherit  Unit=inherit  AffineConversion=off
  SPS Q_j2n6s300_joint_1 : nesl_utility/Simulink-PS Converter  PhysicalDomain=network_engine_domain  SubClassName=ps_input  LeftPortType=input  RightPortType=output  PseudoPeriodic=off  Frequencies=[]  NoiseDistribution=none  NoiseParameters=[]  Unit=1  AffineConversion=off  FilteringAndDerivatives=provide  SimscapeFilterOrder=1  InputFilterTimeConstant=0.001  UdotUserProvided=2
  j2n6s300_joint_1 : sm_lib/Joints/Revolute Joint  JointMode=Normal  SenseConstraintForce=off  SenseConstraintForceX=off  SenseConstraintForceY=off  SenseConstraintForceZ=off  SenseConstraintTorque=off  SenseConstraintTorqueX=off  SenseConstraintTorqueY=off  SenseConstraintTorqueZ=off  SenseTotalForce=off  SenseTotalForceX=off  SenseTotalForceY=off  SenseTotalForceZ=off  SenseTotalTorque=off  SenseTotalTorqueX=off  SenseTotalTorqueY=off  SenseTotalTorqueZ=off  CompositeWrenchDir=FollowerOnBase  CompositeWrenchFrame=BaseFrame  EquilibriumPosition=0  EquilibriumPositionUnits=deg  SpringStiffness=0  SpringStiffnessUnits=N*m/deg  DampingCoefficient=0  DampingCoefficientUnits=kg*m^2/(rad*s)  TorqueActuationMode=ComputedTorque  MotionActuationMode=InputMotion  SensePosition=off  SenseVelocity=off  SenseAcceleration=off  SenseTorqueForce=on  SenseLowerLimitTorqueForce=off  SenseUpperLimitTorqueForce=off  LowerLimitSpecify=off  LowerLimitBound=-90  LowerLimitBoundUnits=deg  LowerLimitStiffness=1e4  LowerLimitStiffnessUnits=N*m/deg  LowerLimitDamping=10  LowerLimitDampingUnits=N*m/(deg/s)  LowerLimitTransitionRegionWidth=0.1  LowerLimitTransitionRegionWidthUnits=deg  UpperLimitSpecify=off  UpperLimitBound=90  UpperLimitBoundUnits=deg  UpperLimitStiffness=1e4  UpperLimitStiffnessUnits=N*m/deg  UpperLimitDamping=10  UpperLimitDampingUnits=N*m/(deg/s)  UpperLimitTransitionRegionWidth=0.1  UpperLimitTransitionRegionWidthUnits=deg  PositionTargetSpecify=on  PositionTargetPriority=High  PositionTargetValue=q0(1)  PositionTargetValueUnits=rad  VelocityTargetSpecify=on  VelocityTargetPriority=High  VelocityTargetValue=dq0(1)  VelocityTargetValueUnits=rad/s
  j2n6s300_link_1 : Subsystem
  Robot Arm : PMIOPort  Side=Right
  Robot Base : PMIOPort  Port=2  Side=Left
  tag scope: Tq_Joint_1=global
  wires:
  [Qddot_Joint_1] -> SPS Q_j2n6s300_joint_1/3
  PSS t_j2n6s300_joint_1/1 -> [Tq_Joint_1]
  [Q_Joint_1] -> SPS Q_j2n6s300_joint_1/1
  [Qdot_Joint_1] -> SPS Q_j2n6s300_joint_1/2
  connections:
  j2n6s300_joint_1/LConn1 -- Robot Base/RConn1
  SPS Q_j2n6s300_joint_1/RConn1 -- j2n6s300_joint_1/LConn2
  j2n6s300_joint_1/RConn1 -- j2n6s300_link_1/LConn1
  j2n6s300_joint_1/RConn2 -- PSS t_j2n6s300_joint_1/LConn1
  Robot Arm/RConn1 -- j2n6s300_link_1/RConn1

== system ManipulatorTrajectoryPlanning_Randomized/Kinova 6DOF Robot Model/Robot Wrist 1 ==
  PSS t_j2n6s300_joint_4 : nesl_utility/PS-Simulink Converter  PhysicalDomain=network_engine_domain  SubClassName=ps_output  LeftPortType=input  RightPortType=output  PseudoPeriodic=off  Frequencies=[]  VectorFormat=inherit  Unit=inherit  AffineConversion=off
  SPS Q_j2n6s300_joint_4 : nesl_utility/Simulink-PS Converter  PhysicalDomain=network_engine_domain  SubClassName=ps_input  LeftPortType=input  RightPortType=output  PseudoPeriodic=off  Frequencies=[]  NoiseDistribution=none  NoiseParameters=[]  Unit=1  AffineConversion=off  FilteringAndDerivatives=provide  SimscapeFilterOrder=1  InputFilterTimeConstant=0.001  UdotUserProvided=2
  j2n6s300_joint_4 : sm_lib/Joints/Revolute Joint  JointMode=Normal  SenseConstraintForce=off  SenseConstraintForceX=off  SenseConstraintForceY=off  SenseConstraintForceZ=off  SenseConstraintTorque=off  SenseConstraintTorqueX=off  SenseConstraintTorqueY=off  SenseConstraintTorqueZ=off  SenseTotalForce=off  SenseTotalForceX=off  SenseTotalForceY=off  SenseTotalForceZ=off  SenseTotalTorque=off  SenseTotalTorqueX=off  SenseTotalTorqueY=off  SenseTotalTorqueZ=off  CompositeWrenchDir=FollowerOnBase  CompositeWrenchFrame=BaseFrame  EquilibriumPosition=0  EquilibriumPositionUnits=deg  SpringStiffness=0  SpringStiffnessUnits=N*m/deg  DampingCoefficient=0  DampingCoefficientUnits=kg*m^2/(rad*s)  TorqueActuationMode=ComputedTorque  MotionActuationMode=InputMotion  SensePosition=off  SenseVelocity=off  SenseAcceleration=off  SenseTorqueForce=on  SenseLowerLimitTorqueForce=off  SenseUpperLimitTorqueForce=off  LowerLimitSpecify=off  LowerLimitBound=-90  LowerLimitBoundUnits=deg  LowerLimitStiffness=1e4  LowerLimitStiffnessUnits=N*m/deg  LowerLimitDamping=10  LowerLimitDampingUnits=N*m/(deg/s)  LowerLimitTransitionRegionWidth=0.1  LowerLimitTransitionRegionWidthUnits=deg  UpperLimitSpecify=off  UpperLimitBound=90  UpperLimitBoundUnits=deg  UpperLimitStiffness=1e4  UpperLimitStiffnessUnits=N*m/deg  UpperLimitDamping=10  UpperLimitDampingUnits=N*m/(deg/s)  UpperLimitTransitionRegionWidth=0.1  UpperLimitTransitionRegionWidthUnits=deg  PositionTargetSpecify=on  PositionTargetPriority=High  PositionTargetValue=q0(4)  PositionTargetValueUnits=rad  VelocityTargetSpecify=on  VelocityTargetPriority=High  VelocityTargetValue=dq0(4)  VelocityTargetValueUnits=rad/s
  j2n6s300_link_4 : Subsystem
  Robot Wrist 2 : PMIOPort  Side=Right
  Robot Forearm : PMIOPort  Port=2  Side=Left
  tag scope: Tq_Joint_4=global
  wires:
  PSS t_j2n6s300_joint_4/1 -> [Tq_Joint_4]
  [Qddot_Joint_4] -> SPS Q_j2n6s300_joint_4/3
  [Q_Joint_4] -> SPS Q_j2n6s300_joint_4/1
  [Qdot_Joint_4] -> SPS Q_j2n6s300_joint_4/2
  connections:
  Robot Wrist 2/RConn1 -- j2n6s300_link_4/RConn1
  j2n6s300_joint_4/RConn2 -- PSS t_j2n6s300_joint_4/LConn1
  j2n6s300_joint_4/RConn1 -- j2n6s300_link_4/LConn1
  SPS Q_j2n6s300_joint_4/RConn1 -- j2n6s300_joint_4/LConn2
  j2n6s300_joint_4/LConn1 -- Robot Forearm/RConn1

== system ManipulatorTrajectoryPlanning_Randomized/Kinova 6DOF Robot Model/Robot Wrist 2 ==
  PSS t_j2n6s300_joint_5 : nesl_utility/PS-Simulink Converter  PhysicalDomain=network_engine_domain  SubClassName=ps_output  LeftPortType=input  RightPortType=output  PseudoPeriodic=off  Frequencies=[]  VectorFormat=inherit  Unit=inherit  AffineConversion=off
  SPS Q_j2n6s300_joint_5 : nesl_utility/Simulink-PS Converter  PhysicalDomain=network_engine_domain  SubClassName=ps_input  LeftPortType=input  RightPortType=output  PseudoPeriodic=off  Frequencies=[]  NoiseDistribution=none  NoiseParameters=[]  Unit=1  AffineConversion=off  FilteringAndDerivatives=provide  SimscapeFilterOrder=1  InputFilterTimeConstant=0.001  UdotUserProvided=2
  j2n6s300_joint_5 : sm_lib/Joints/Revolute Joint  JointMode=Normal  SenseConstraintForce=off  SenseConstraintForceX=off  SenseConstraintForceY=off  SenseConstraintForceZ=off  SenseConstraintTorque=off  SenseConstraintTorqueX=off  SenseConstraintTorqueY=off  SenseConstraintTorqueZ=off  SenseTotalForce=off  SenseTotalForceX=off  SenseTotalForceY=off  SenseTotalForceZ=off  SenseTotalTorque=off  SenseTotalTorqueX=off  SenseTotalTorqueY=off  SenseTotalTorqueZ=off  CompositeWrenchDir=FollowerOnBase  CompositeWrenchFrame=BaseFrame  EquilibriumPosition=0  EquilibriumPositionUnits=deg  SpringStiffness=0  SpringStiffnessUnits=N*m/deg  DampingCoefficient=0  DampingCoefficientUnits=kg*m^2/(rad*s)  TorqueActuationMode=ComputedTorque  MotionActuationMode=InputMotion  SensePosition=off  SenseVelocity=off  SenseAcceleration=off  SenseTorqueForce=on  SenseLowerLimitTorqueForce=off  SenseUpperLimitTorqueForce=off  LowerLimitSpecify=off  LowerLimitBound=-90  LowerLimitBoundUnits=deg  LowerLimitStiffness=1e4  LowerLimitStiffnessUnits=N*m/deg  LowerLimitDamping=10  LowerLimitDampingUnits=N*m/(deg/s)  LowerLimitTransitionRegionWidth=0.1  LowerLimitTransitionRegionWidthUnits=deg  UpperLimitSpecify=off  UpperLimitBound=90  UpperLimitBoundUnits=deg  UpperLimitStiffness=1e4  UpperLimitStiffnessUnits=N*m/deg  UpperLimitDamping=10  UpperLimitDampingUnits=N*m/(deg/s)  UpperLimitTransitionRegionWidth=0.1  UpperLimitTransitionRegionWidthUnits=deg  PositionTargetSpecify=on  PositionTargetPriority=High  PositionTargetValue=q0(5)  PositionTargetValueUnits=rad  VelocityTargetSpecify=on  VelocityTargetPriority=High  VelocityTargetValue=dq0(5)  VelocityTargetValueUnits=rad/s
  j2n6s300_link_5 : Subsystem
  Robot End Effector : PMIOPort  Side=Right
  Robot Wrist 1 : PMIOPort  Port=2  Side=Left
  tag scope: Tq_Joint_5=global
  wires:
  [Qdot_Joint_5] -> SPS Q_j2n6s300_joint_5/2
  PSS t_j2n6s300_joint_5/1 -> [Tq_Joint_5]
  [Qddot_Joint_5] -> SPS Q_j2n6s300_joint_5/3
  [Q_Joint_5] -> SPS Q_j2n6s300_joint_5/1
  connections:
  SPS Q_j2n6s300_joint_5/RConn1 -- j2n6s300_joint_5/LConn2
  Robot End Effector/RConn1 -- j2n6s300_link_5/RConn1
  j2n6s300_joint_5/RConn1 -- j2n6s300_link_5/LConn1
  j2n6s300_joint_5/LConn1 -- Robot Wrist 1/RConn1
  j2n6s300_joint_5/RConn2 -- PSS t_j2n6s300_joint_5/LConn1

== system ManipulatorTrajectoryPlanning_Randomized/Kinova 6DOF Robot Model/j2n6s300_end_effector ==
  Inertia : sm_lib/Body Elements/Inertia  InertiaType=Custom  Mass=0  MassUnits=kg  CenterOfMass=[0, 0, 0]  CenterOfMassUnits=m  MomentsOfInertia=[0, 0, 0]  MomentsOfInertiaUnits=kg*m^2  ProductsOfInertia=[0, 0, 0]  ProductsOfInertiaUnits=kg*m^2  GraphicType=None  MarkerShape=Inertia  MarkerSize=20  GraphicVisPropType=SimpleVisualProperties  GraphicDiffuseColor=[0.5 0.5 0.5]  GraphicSpecularColor=[0.5 0.5 0.5 1.0]  GraphicAmbientColor=[0.15 0.15 0.15 1.0]  GraphicEmissiveColor=[0.0 0.0 0.0 1.0]  GraphicShininess=75  GraphicOpacity=1.0
  InertiaOriginTransform : sm_lib/Frames and Transforms/Rigid Transform  TranslationMethod=Cartesian  TranslationStandardOffset=0  TranslationLengthUnit=m  TranslationStandardAxis=+Z  TranslationCartesianOffset=[0, 0, 0]  TranslationROffset=0  TranslationROffsetUnits=m  TranslationZOffset=0  TranslationZOffsetUnits=m  TranslationThetaOffset=0  TranslationThetaOffsetUnits=deg  RotationMethod=RotationSequence  RotationAngleUnits=deg  RotationStandardAxis=+Z  RotationAngle=0.0  RotationArbitraryAxis=[0 0 1]  FollAlignAxisA=+X  BaseAlignAxisA=+Y  FollAlignAxisB=+Y  BaseAlignAxisB=+Z  RotationSequenceAxes=BaseAxes  RotationSequence=XYZ  RotationSequenceAngles=[0, 0, 0]  RotationSequenceAnglesUnits=rad  RotationMatrix=[1 0 0; 0 1 0; 0 0 1]  Quaternion=[1 0 0 0]
  ReferenceFrame : sm_lib/Frames and Transforms/Reference Frame
  Visual : sm_lib/Body Elements/Brick Solid  GraphicAmbientColor=[0.15 0.15 0.15 1.0]  BasedOnType=Density  BrickDimensions=[0.001, 0.001, 0.001]  BrickDimensionUnits=m  CenterOfMass=[0, 0, 0]  CenterOfMassUnits=m  GraphicDiffuseColor=[0.5, 0.5, 0.5]  Density=1000  DensityUnits=kg/m^3  DoExposeReferenceFrame=on  GraphicEmissiveColor=[0.0 0.0 0.0 1.0]  ExportEntireGeometry=off  SerializedFrames=<Frames><Frame><Id>Frame1</Id><Value><Name>F1</Name><Origin><Source>GeometricFeature</Source><FeatureName>-z surface</FeatureName></Origin><PrimaryAxis><DefinedDirection>+Z</DefinedDirection><Source>ReferenceFrame</Source><SourceDirection>+Z</SourceDirection><FeatureName></FeatureName></PrimaryAxis><SecondaryAxis><DefinedDirection>+X</DefinedDirection><Source>ReferenceFrame</Source><SourceDirection>+X</SourceDirection><FeatureName></FeatureName></SecondaryAxis></Value></Frame></Frames>  MarkerShape=Sphere  MarkerSize=10  GraphicType=FromGeometry  InertiaType=Custom  Mass=0  MassUnits=kg  MomentsOfInertia=[0, 0, 0]  MomentsOfInertiaUnits=kg*m^2  GraphicOpacity=1  ProductsOfInertia=[0, 0, 0]  ProductsOfInertiaUnits=kg*m^2  GraphicShininess=75  GraphicSpecularColor=[0.5 0.5 0.5 1.0]  GraphicVisPropType=SimpleVisualProperties
  VisualOriginTransform : sm_lib/Frames and Transforms/Rigid Transform  TranslationMethod=Cartesian  TranslationStandardOffset=0  TranslationLengthUnit=m  TranslationStandardAxis=+Z  TranslationCartesianOffset=[0, 0, 0]  TranslationROffset=0  TranslationROffsetUnits=m  TranslationZOffset=0  TranslationZOffsetUnits=m  TranslationThetaOffset=0  TranslationThetaOffsetUnits=deg  RotationMethod=RotationSequence  RotationAngleUnits=deg  RotationStandardAxis=+Z  RotationAngle=0.0  RotationArbitraryAxis=[0 0 1]  FollAlignAxisA=+X  BaseAlignAxisA=+Y  FollAlignAxisB=+Y  BaseAlignAxisB=+Z  RotationSequenceAxes=BaseAxes  RotationSequence=XYZ  RotationSequenceAngles=[0, 0, 0]  RotationSequenceAnglesUnits=rad  RotationMatrix=[1 0 0; 0 1 0; 0 0 1]  Quaternion=[1 0 0 0]
  F : PMIOPort  Side=Left
  R : PMIOPort  Port=2  Side=Right
  connections:
  Inertia/RConn1 -- InertiaOriginTransform/RConn1
  ReferenceFrame/RConn1 -- InertiaOriginTransform/LConn1 -- VisualOriginTransform/LConn1 -- F/RConn1
  VisualOriginTransform/RConn1 -- Visual/LConn1
  R/RConn1 -- Visual/RConn1
